simulink model "a2"  (R2016a)
settings: Solver=VariableStepAuto  StartTime=0.0  StopTime=100.0  RelTol=1e-3
values from neighbouring files (symbols this model uses):
  n = n+1    (= 1)    [Erlang_Fixed_Point_Method.m]
undefined symbols (not defined in the file or in its folder): m
libraries: simulink x2
settings Model: Creator=s168877  LastModifiedBy=s168877

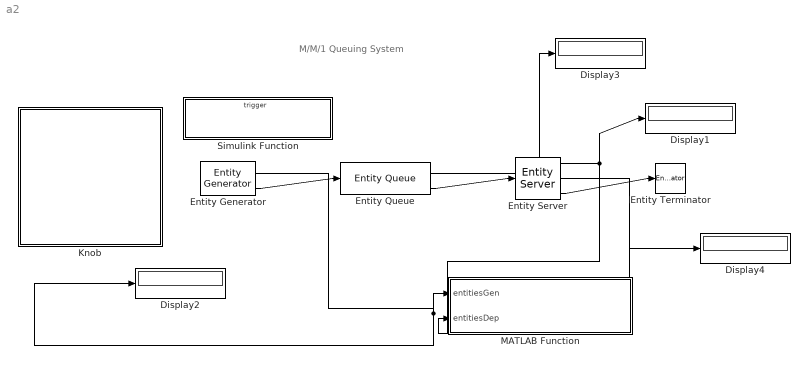
== system a2 ==
  note: M/M/1 Queuing System
  Display{1..4} (4 alike) : Display
  Entity Generator : EntityGenerator  OutputPortMessageModes=n,m  TimeSource=MATLAB action  IntergenerationTimeAction=dt = exponentialArrivalTime1();  AttributeName=Class  NumberEntitiesDeparted=on  EntityType=Structured  EntityTypeName=Entity
      settings: OutputPortMap=o0,o3
  Entity Queue : EntityQueue  InputPortMessageModes=m  OutputPortMessageModes=n,m  Capacity=Inf  NumberEntitiesInBlock=on
      settings: OutputPortMap=o1,o5
  Entity Server : EntityServer  InputPortMessageModes=m  OutputPortMessageModes=n,n,m  Capacity=N  ServiceTimeSource=MATLAB action  ServiceTimeAction=|  NumberEntitiesDeparted=on  NumberEntitiesInBlock=on
      | % Exponential service time with rate 1
      | mean = computemean(1);
      | dt   = -mean * log(1 - rand());
      settings: OutputPortMap=o0,o1,o9
  Entity Terminator : EntityTerminator  InputPortMessageModes=m
  Knob : Subsystem  DialogController=hmiCreateDDGDialog  IsWebBlock=on  mask(MWDashboardBlock){webBlockId=c16762df-0ec6-45f2-8822-9c3d7e5a9624, webBlockType=continuousknob, ShowInLibBrowser=on, ShowInitialText=on, HMISrcModelName=a2}
      mask prompts: webBlockId "WebBlock Id"; webBlockType "WebBlock Type"; HMISrcModelName "Source Model"
      mask Help: helpview([docroot '/mapfiles/simulink.map'], 'hmi_knob')
      mask Display:
      | if strcmp(get_param(bdroot(gcb),'BlockDiagramType'), 'library')
      |     image([(matlabroot) '/toolbox/simulink/hmi/icons/ContinuousKnob.png']);
      | end
  MATLAB Function : MATLAB Function  TreatAsAtomicUnit=on
  Simulink Function : Subsystem  TreatAsAtomicUnit=on
  wires:
  Entity Generator/2 -> Entity Queue/1
  Entity Queue/2 -> Entity Server/1
  Entity Server/3 -> Entity Terminator/1
  Entity Server/1 -> MATLAB Function/2(entitiesDep), Display1/1
  Entity Generator/1 -> Display2/1, MATLAB Function/1(entitiesGen)
  Entity Queue/1 -> Display3/1
  Entity Server/2 -> Display4/1

== system a2/Knob ==

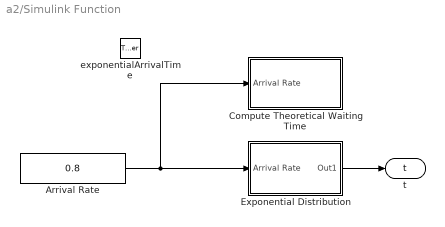
== system a2/Simulink Function ==
  exponentialArrivalTime : TriggerPort  TriggerType=function-call  IsSimulinkFunction=on  FunctionName=exponentialArrivalTime1  VariantControl=Variant
  Arrival Rate : Constant  Value=0.8  SampleTime=-1
  Compute Theoretical Waiting Time : Subsystem
  Exponential Distribution : Subsystem
  t : ArgOut  DisableCoverage=on  ArgumentName=t
  wires:
  Arrival Rate/1 -> Compute Theoretical Waiting Time/1(Arrival Rate), Exponential Distribution/1(Arrival Rate)
  Exponential Distribution/1(Out1) -> t/1

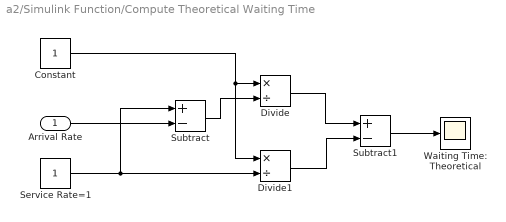
== system a2/Simulink Function/Compute Theoretical Waiting Time ==
  Arrival Rate : Inport
  Constant : Constant
  Divide : Product  Inputs=*/
  Divide1 : Product  Inputs=*/
  Service Rate=1 : Constant
  Subtract : Sum  Inputs=+-
  Subtract1 : Sum  Inputs=+-
  Waiting Time: Theoretical : Scope
  wires:
  Arrival Rate/1 -> Subtract/2
  Subtract1/1 -> Waiting Time: Theoretical/1
  Divide1/1 -> Subtract1/2
  Divide/1 -> Subtract1/1
  Subtract/1 -> Divide/2
  Constant/1 -> Divide1/1, Divide/1
  Service Rate=1/1 -> Subtract/1, Divide1/2

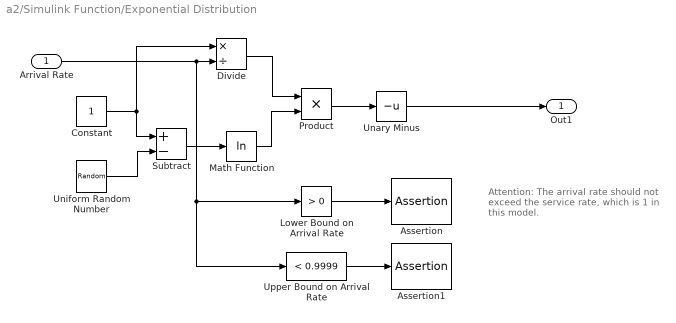
== system a2/Simulink Function/Exponential Distribution ==
  note: Attention: The arrival rate
      | should not exceed the service
      | rate, which is 1 in this model.
  Arrival Rate : Inport
  Assertion : Assertion
  Assertion1 : Assertion
  Constant : Constant
  Divide : Product  Inputs=*/
  Lower Bound on Arrival Rate : simulink/Logic and Bit Operations/Compare To Constant  relop=>  const=0  OutDataTypeStr=uint8  ZeroCross=off
  Math Function : Math  Operator=log  SaturateOnIntegerOverflow=on
  Product : Product  RndMeth=Zero
  Subtract : Sum  Inputs=+-
  Unary Minus : UnaryMinus
  Uniform Random Number : UniformRandomNumber  Minimum=0  Seed=12345
  "Upper Bound on Arrival Rate " : simulink/Logic and Bit Operations/Compare To Constant  relop=<  const=0.9999  OutDataTypeStr=uint8  ZeroCross=off
  Out1 : Outport
  wires:
  Arrival Rate/1 -> Divide/2, Lower Bound on Arrival Rate/1, "Upper Bound on Arrival Rate "/1
  Unary Minus/1 -> Out1/1
  Product/1 -> Unary Minus/1
  Math Function/1 -> Product/2
  Divide/1 -> Product/1
  Constant/1 -> Divide/1, Subtract/1
  Uniform Random Number/1 -> Subtract/2
  Lower Bound on Arrival Rate/1 -> Assertion/1
  "Upper Bound on Arrival Rate "/1 -> Assertion1/1
  Subtract/1 -> Math Function/1

== matlab function a2/MATLAB Function ==
  data: entitiesGen input; entitiesDep input
function fcn(entitiesGen,entitiesDep)
%#codegen
coder.extrinsic('assignin');
entitiesInsys=entitiesGen-entitiesDep;
assignin('base','N',entitiesInsys);

end
